simulink model "is_sim"  (R2025b)
settings: Solver=VariableStepAuto  StartTime=0.0  StopTime=10.0  RelTol=1e-3
libraries: simulink x4
settings Model: Creator=David  LastModifiedBy=David

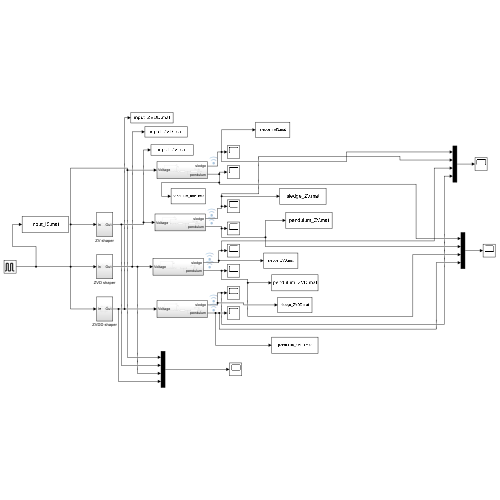
[thumbnail: Simulink's stored preview of the top-level diagram]
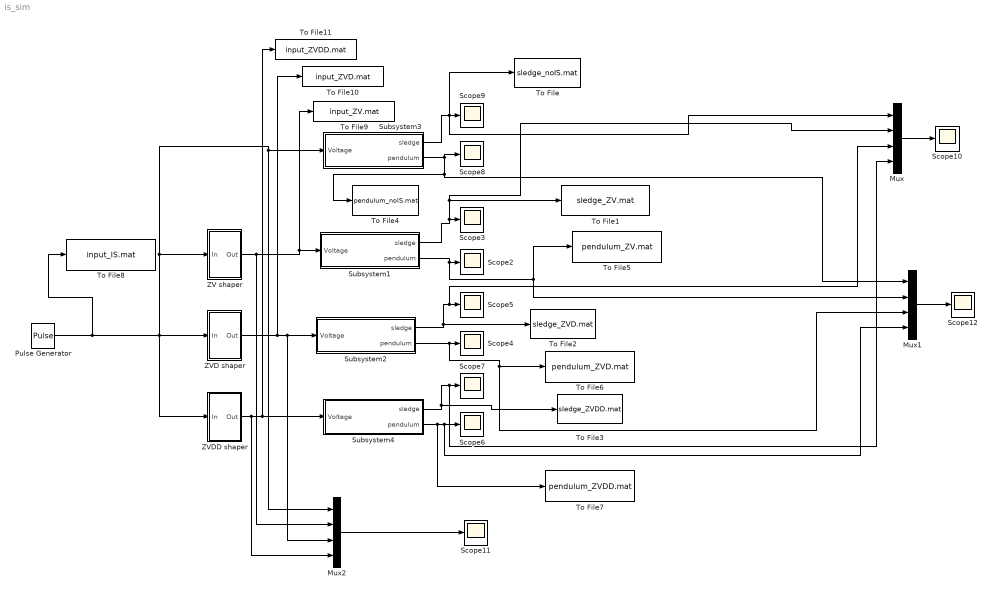
== system is_sim ==
  Mux : Mux
  Mux1 : Mux
  Mux2 : Mux
  Pulse Generator : DiscretePulseGenerator  PulseType=Time based  Amplitude=4  Period=50  PulseWidth=5  PhaseDelay=2
  Scope{2..12} (11 alike) : Scope
      Scope10 settings: ActiveDisplayYMinimum=-1  ActiveDisplayYMaximum=1  DataLoggingVariableName=ScopeData11
      Scope11 settings: ActiveDisplayYMinimum=-1  ActiveDisplayYMaximum=1  DataLoggingVariableName=ScopeData14
      Scope12 settings: ActiveDisplayYMinimum=-0.19127007055974196  ActiveDisplayYMaximum=0.19414151473599317  DataLoggingVariableName=ScopeData12
      Scope2 settings: ActiveDisplayYMinimum=-1  ActiveDisplayYMaximum=1  DataLoggingVariableName=ScopeData13
      Scope3 settings: ActiveDisplayYMinimum=-1  ActiveDisplayYMaximum=1  DataLoggingVariableName=ScopeData3
      Scope4 settings: ActiveDisplayYMinimum=-0.16064529340853845  ActiveDisplayYMaximum=0.1569195069828942  DataLoggingVariableName=ScopeData4
      Scope5 settings: ActiveDisplayYMinimum=-1  ActiveDisplayYMaximum=1  DataLoggingVariableName=ScopeData5
      Scope6 settings: ActiveDisplayYMinimum=-0.031481974632713523  ActiveDisplayYMaximum=0.031767037821901635  DataLoggingVariableName=ScopeData6
      Scope7 settings: ActiveDisplayYMinimum=-1  ActiveDisplayYMaximum=1  DataLoggingVariableName=ScopeData7
      Scope8 settings: ActiveDisplayYMinimum=-1  ActiveDisplayYMaximum=1  DataLoggingVariableName=ScopeData8
      Scope9 settings: ActiveDisplayYMinimum=-1  ActiveDisplayYMaximum=1  DataLoggingVariableName=ScopeData9
  Subsystem1 : Subsystem
  Subsystem2 : Subsystem
  Subsystem3 : Subsystem
  Subsystem4 : Subsystem
  To File : ToFile  Filename=sledge_noIS.mat  SaveFormat=Timeseries
  To File1 : ToFile  Filename=sledge_ZV.mat  SaveFormat=Timeseries
  To File10 : ToFile  Filename=input_ZVD.mat  SaveFormat=Timeseries
  To File11 : ToFile  Filename=input_ZVDD.mat  SaveFormat=Timeseries
  To File2 : ToFile  Filename=sledge_ZVD.mat  SaveFormat=Timeseries
  To File3 : ToFile  Filename=sledge_ZVDD.mat  SaveFormat=Timeseries
  To File4 : ToFile  Filename=pendulum_noIS.mat  SaveFormat=Timeseries
  To File5 : ToFile  Filename=pendulum_ZV.mat  SaveFormat=Timeseries
  To File6 : ToFile  Filename=pendulum_ZVD.mat  SaveFormat=Timeseries
  To File7 : ToFile  Filename=pendulum_ZVDD.mat  SaveFormat=Timeseries
  To File8 : ToFile  Filename=input_IS.mat  SaveFormat=Timeseries
  To File9 : ToFile  Filename=input_ZV.mat  SaveFormat=Timeseries
  ZV shaper : Subsystem
  ZVD shaper : Subsystem
  ZVDD shaper : Subsystem
  wires:
  Subsystem2/1(sledge) -> Mux/3, Scope5/1, To File2/1
  ZV shaper/1(Out) -> Mux2/2, Subsystem1/1(Voltage), To File9/1
  Mux2/1 -> Scope11/1
  Subsystem2/2(pendulum) -> Mux1/3, To File6/1, Scope4/1
  Mux1/1 -> Scope12/1
  Subsystem4/2(pendulum) -> To File7/1, Mux1/4, Scope6/1
  Subsystem1/2(pendulum) -> To File5/1, Mux1/2, Scope2/1
  Subsystem3/2(pendulum) -> Scope8/1, Mux1/1, To File4/1
  Mux/1 -> Scope10/1
  ZVD shaper/1(Out) -> To File10/1, Subsystem2/1(Voltage), Mux2/3
  Subsystem3/1(sledge) -> To File/1, Mux/1, Scope9/1
  Subsystem1/1(sledge) -> Mux/2, To File1/1, Scope3/1
  Subsystem4/1(sledge) -> Mux/4, Scope7/1, To File3/1
  Pulse Generator/1 -> To File8/1, ZVDD shaper/1(In), Subsystem3/1(Voltage), Mux2/1, ZV shaper/1(In), ZVD shaper/1(In)
  ZVDD shaper/1(Out) -> Mux2/4, Subsystem4/1(Voltage), To File11/1

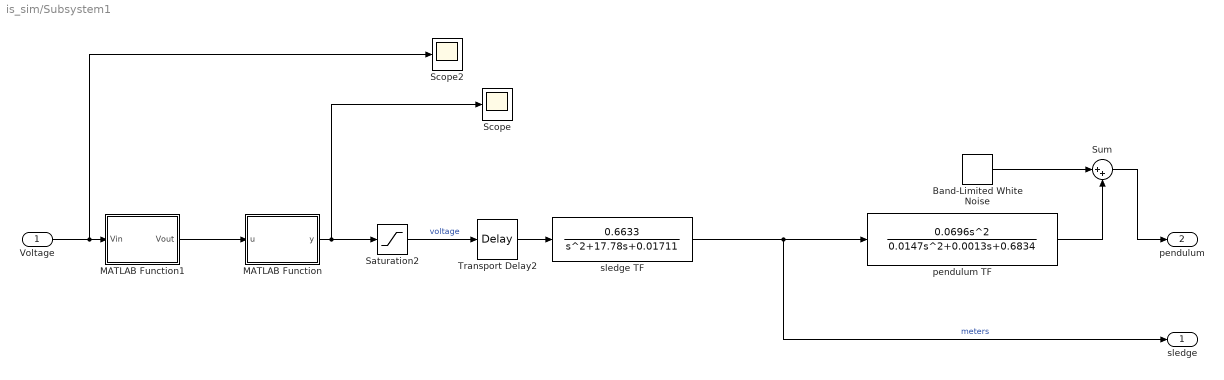
== system is_sim/Subsystem1 ==
  Voltage : Inport
  Band-Limited White Noise : simulink/Sources/Band-Limited White Noise  Cov=[4.9008e-09]  Ts=0.01  seed=[23341]
  MATLAB Function : MATLAB Function  TreatAsAtomicUnit=on
  MATLAB Function1 : MATLAB Function  TreatAsAtomicUnit=on
  Saturation2 : Saturate  UpperLimit=16  LowerLimit=-16
  Scope : Scope
      settings: ActiveDisplayYMinimum=-1  ActiveDisplayYMaximum=1
  Scope2 : Scope
      settings: ActiveDisplayYMinimum=-1  ActiveDisplayYMaximum=1  DataLoggingVariableName=ScopeData10
  Sum : Sum  Inputs=|++
  Transport Delay2 : TransportDelay  DelayTime=0.01
  pendulum TF : TransferFcn  Numerator=[0.0696 0 0]  Denominator=[0.0147 0.0013 0.6834]
  sledge TF : TransferFcn  Numerator=0.6633  Denominator=[1 17.78 0.01711]
  sledge : Outport
  pendulum : Outport  Port=2
  wires:
  Saturation2/1 -> Transport Delay2/1  "voltage"
  sledge TF/1 -> pendulum TF/1, sledge/1  "meters"
  pendulum TF/1 -> Sum/2
  Band-Limited White Noise/1 -> Sum/1
  Sum/1 -> pendulum/1
  Voltage/1 -> MATLAB Function1/1(Vin), Scope2/1
  MATLAB Function1/1(Vout) -> MATLAB Function/1(u)
  MATLAB Function/1(y) -> Scope/1, Saturation2/1
  Transport Delay2/1 -> sledge TF/1

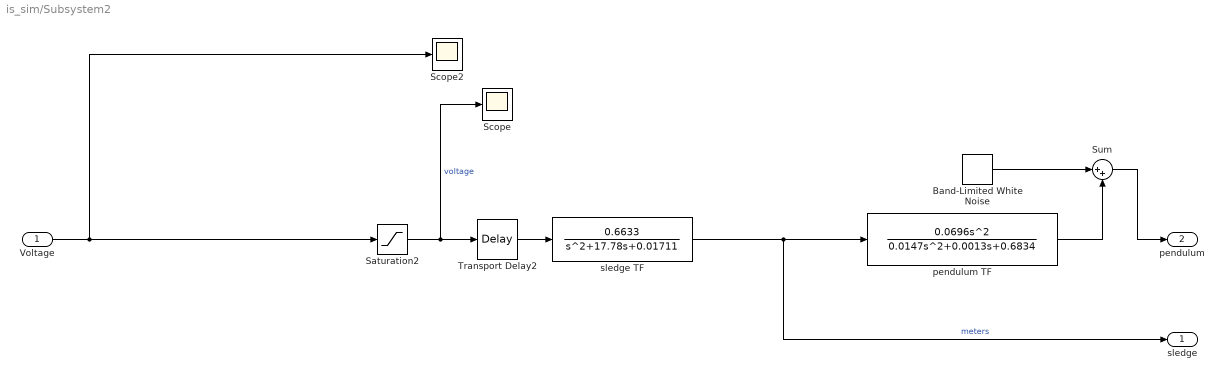
== system is_sim/Subsystem2 ==
  Voltage : Inport
  Band-Limited White Noise : simulink/Sources/Band-Limited White Noise  Cov=[4.9008e-09]  Ts=0.01  seed=[23341]
  Saturation2 : Saturate  UpperLimit=16  LowerLimit=-16
  Scope : Scope
      settings: ActiveDisplayYMinimum=-1  ActiveDisplayYMaximum=1
  Scope2 : Scope
      settings: ActiveDisplayYMinimum=-1  ActiveDisplayYMaximum=1  DataLoggingVariableName=ScopeData10
  Sum : Sum  Inputs=|++
  Transport Delay2 : TransportDelay  DelayTime=0.01
  pendulum TF : TransferFcn  Numerator=[0.0696 0 0]  Denominator=[0.0147 0.0013 0.6834]
  sledge TF : TransferFcn  Numerator=0.6633  Denominator=[1 17.78 0.01711]
  sledge : Outport
  pendulum : Outport  Port=2
  wires:
  Saturation2/1 -> Transport Delay2/1, Scope/1  "voltage"
  sledge TF/1 -> pendulum TF/1, sledge/1  "meters"
  pendulum TF/1 -> Sum/2
  Band-Limited White Noise/1 -> Sum/1
  Sum/1 -> pendulum/1
  Voltage/1 -> Saturation2/1, Scope2/1
  Transport Delay2/1 -> sledge TF/1

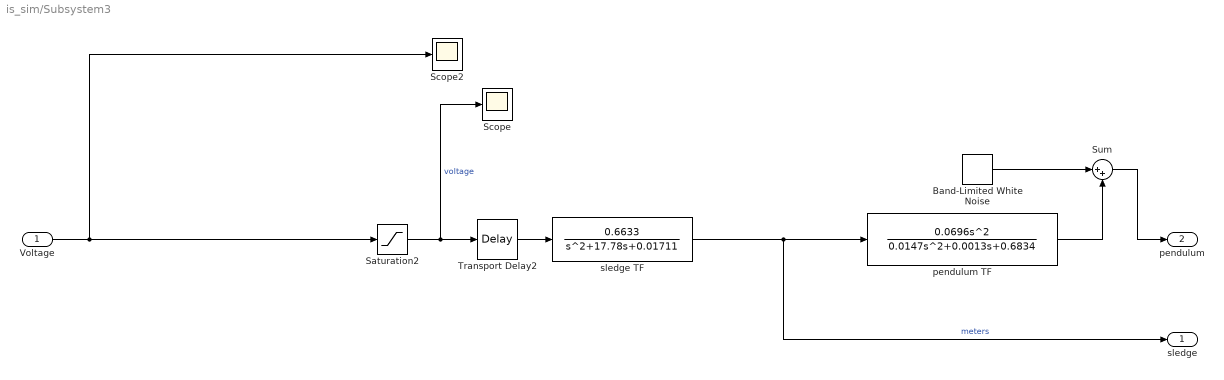
== system is_sim/Subsystem3 ==
  Voltage : Inport
  Band-Limited White Noise : simulink/Sources/Band-Limited White Noise  Cov=[4.9008e-09]  Ts=0.01  seed=[23341]
  Saturation2 : Saturate  UpperLimit=16  LowerLimit=-16
  Scope : Scope
      settings: ActiveDisplayYMinimum=-1  ActiveDisplayYMaximum=1
  Scope2 : Scope
      settings: ActiveDisplayYMinimum=-1  ActiveDisplayYMaximum=1  DataLoggingVariableName=ScopeData10
  Sum : Sum  Inputs=|++
  Transport Delay2 : TransportDelay  DelayTime=0.01
  pendulum TF : TransferFcn  Numerator=[0.0696 0 0]  Denominator=[0.0147 0.0013 0.6834]
  sledge TF : TransferFcn  Numerator=0.6633  Denominator=[1 17.78 0.01711]
  sledge : Outport
  pendulum : Outport  Port=2
  wires:
  Saturation2/1 -> Transport Delay2/1, Scope/1  "voltage"
  sledge TF/1 -> pendulum TF/1, sledge/1  "meters"
  pendulum TF/1 -> Sum/2
  Band-Limited White Noise/1 -> Sum/1
  Sum/1 -> pendulum/1
  Voltage/1 -> Saturation2/1, Scope2/1
  Transport Delay2/1 -> sledge TF/1

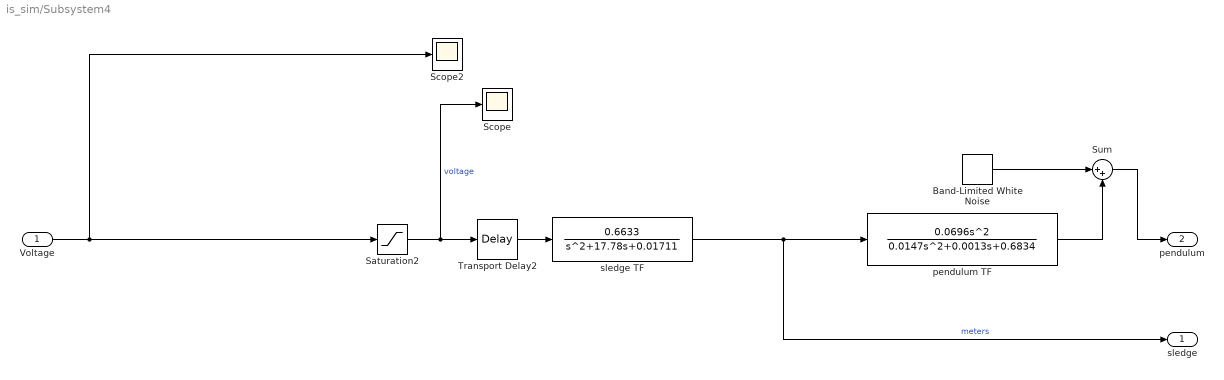
== system is_sim/Subsystem4 ==
  Voltage : Inport
  Band-Limited White Noise : simulink/Sources/Band-Limited White Noise  Cov=[4.9008e-09]  Ts=0.01  seed=[23341]
  Saturation2 : Saturate  UpperLimit=16  LowerLimit=-16
  Scope : Scope
      settings: ActiveDisplayYMinimum=-1  ActiveDisplayYMaximum=1
  Scope2 : Scope
      settings: ActiveDisplayYMinimum=-1  ActiveDisplayYMaximum=1  DataLoggingVariableName=ScopeData10
  Sum : Sum  Inputs=|++
  Transport Delay2 : TransportDelay  DelayTime=0.01
  pendulum TF : TransferFcn  Numerator=[0.0696 0 0]  Denominator=[0.0147 0.0013 0.6834]
  sledge TF : TransferFcn  Numerator=0.6633  Denominator=[1 17.78 0.01711]
  sledge : Outport
  pendulum : Outport  Port=2
  wires:
  Saturation2/1 -> Transport Delay2/1, Scope/1  "voltage"
  sledge TF/1 -> pendulum TF/1, sledge/1  "meters"
  pendulum TF/1 -> Sum/2
  Band-Limited White Noise/1 -> Sum/1
  Sum/1 -> pendulum/1
  Voltage/1 -> Saturation2/1, Scope2/1
  Transport Delay2/1 -> sledge TF/1

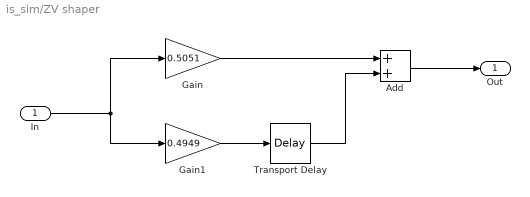
== system is_sim/ZV shaper ==
  In : Inport
  Add : Sum
  Gain : Gain  Gain=0.5051
  Gain1 : Gain  Gain=0.4949
  Transport Delay : TransportDelay  DelayTime=0.4607
  Out : Outport
  wires:
  Add/1 -> Out/1
  In/1 -> Gain/1, Gain1/1
  Gain1/1 -> Transport Delay/1
  Transport Delay/1 -> Add/2
  Gain/1 -> Add/1

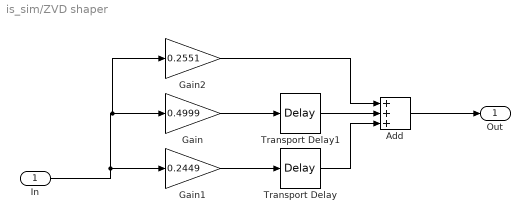
== system is_sim/ZVD shaper ==
  In : Inport
  Add : Sum  Inputs=+++
  Gain : Gain  Gain=0.4999
  Gain1 : Gain  Gain=0.2449
  Gain2 : Gain  Gain=0.2551
  Transport Delay : TransportDelay  DelayTime=0.9215
  Transport Delay1 : TransportDelay  DelayTime=0.4607
  Out : Outport
  wires:
  Gain/1 -> Transport Delay1/1
  Gain1/1 -> Transport Delay/1
  In/1 -> Gain1/1, Gain2/1, Gain/1
  Add/1 -> Out/1
  Transport Delay1/1 -> Add/2
  Transport Delay/1 -> Add/3
  Gain2/1 -> Add/1

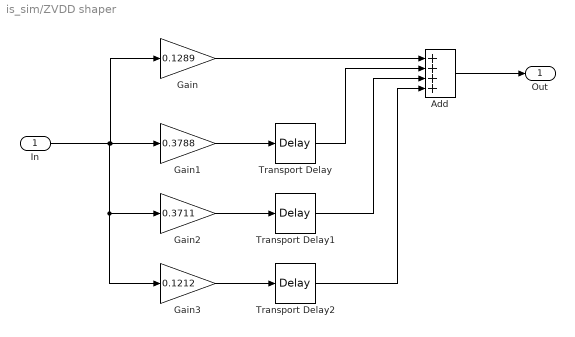
== system is_sim/ZVDD shaper ==
  In : Inport
  Add : Sum  Inputs=++++
  Gain : Gain  Gain=0.1289
  Gain1 : Gain  Gain=0.3788
  Gain2 : Gain  Gain=0.3711
  Gain3 : Gain  Gain=0.1212
  Transport Delay : TransportDelay  DelayTime=0.4607
  Transport Delay1 : TransportDelay  DelayTime=0.9215
  Transport Delay2 : TransportDelay  DelayTime=1.3822
  Out : Outport
  wires:
  Add/1 -> Out/1
  In/1 -> Gain/1, Gain1/1, Gain3/1, Gain2/1
  Gain1/1 -> Transport Delay/1
  Transport Delay/1 -> Add/2
  Gain/1 -> Add/1
  Gain3/1 -> Transport Delay2/1
  Gain2/1 -> Transport Delay1/1
  Transport Delay1/1 -> Add/3
  Transport Delay2/1 -> Add/4

== matlab function is_sim/Subsystem1/MATLAB Function1 ==
  data: Vin input; Vout output
function Vout = mapping(Vin)
V_min = 4.6;
V_max = 24;

Vout = Vin*(V_max - V_min)/(V_max) + V_min;

end

== matlab function is_sim/Subsystem1/MATLAB Function ==
  data: u input; y output
function y = deadzone(u)
V_min = 4.61;

if abs(u) < V_min
    y = 0;
else
    y = u;
end
